simulink model "collectors"  (R2018a)
settings: Solver=VariableStepAuto  StartTime=0.0  StopTime=500  FixedStep=0.01  RelTol=1e-5
libraries: simulink x2
settings Model: Creator=daniel  LastModifiedBy=blond
settings SolverCC: ZeroCrossAlgorithm=Adaptive  AlgebraicLoopSolver=LineSearch
settings DebuggingCC: MaxConsecutiveZCsMsg=warning

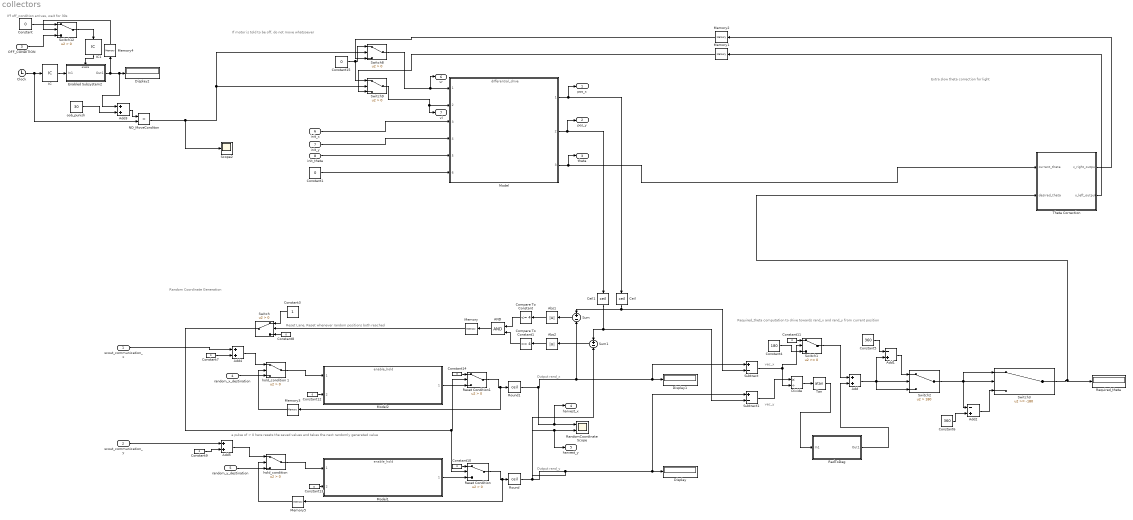
== system collectors ==
  note: If motor is told to be off, do not move whatsoever
  note: Extra slow theta correction for light
  note: Required_theta computation to drive towards rand_x and rand_y from current position
  note: vec_y
  note: Reset Lane, Reset whenever random positions both reached
  note: a pulse of > 0 here resets the saved values and takes the next randomly generated value
  note: Output rand_x
  note: Random Coordinate Generation
  note: Output rand_y
  note: vec_x
  note: Iff off_condition arrives, wait for 30s
  "scout_communication_x " : Inport
  scout_communication_y : Inport  Port=2
  "OFF_CONDITION " : Inport  Port=3  OutDataTypeStr=boolean
  random_x_destination : Inport  Port=4
  random_y_destination : Inport  Port=5
  "init_x " : Inport  Port=6
  init_y : Inport  Port=7
  "init_theta " : Inport  Port=8
  AND : Logic  IconShape=distinctive  AllPortsSameDT=off  OutDataTypeStr=boolean
  Abs1 : Abs
  Abs2 : Abs
  Add{,3..5} (4 alike) : Sum
  Add1 : Sum  Inputs=-+
  Add2 : Sum  Inputs=-+
  Ceil : Rounding  Operator=ceil
  Ceil1 : Rounding  Operator=ceil
  Clock : Clock
  Compare To Constant : simulink/Logic and Bit Operations/Compare To Constant  relop=<=  const=4  OutDataTypeStr=boolean
  Compare To Constant1 : simulink/Logic and Bit Operations/Compare To Constant  relop=<=  const=4  OutDataTypeStr=boolean
  Constant{,1,7..15} (11 alike) : Constant  Value=0
  Constant3 : Constant
  Constant4 : Constant  Value=180
  Constant5 : Constant  Value=360
  Constant6 : Constant  Value=360
  Display : Display
  Display1 : Display
  Display2 : Display
  Divide : Product  Inputs=*/
  Enabled Subsystem2 : Subsystem  TreatAsAtomicUnit=on
  IC : InitialCondition  Value=-30
  IC1 : InitialCondition
  Memory{,1..2,4} (4 alike) : Memory
  Memory3 : Memory  InheritSampleTime=on
  Memory5 : Memory  InheritSampleTime=on
  Model : ModelReference  ModelNameDialog=differential_drive.slx  SimulationMode=Normal  ModelReferenceVersion=1.313
  Model1 : ModelReference  ModelNameDialog=enable_hold.slx  SimulationMode=Normal  ModelReferenceVersion=1.286
  Model2 : ModelReference  ModelNameDialog=enable_hold.slx  SimulationMode=Normal  ModelReferenceVersion=1.286
  NO_MoveConditon : RelationalOperator  Operator=>  OutDataTypeStr=boolean  RndMeth=Simplest
  RadToDeg : Subsystem
  "RandomCoordinate Scope " : Scope  NumInputPorts=2
  Required_theta : Display
  Reset Condition : Switch  Criteria=u2 > Threshold
  Reset Condition1 : Switch  Criteria=u2 > Threshold
  Round : Rounding  Operator=ceil
  Round1 : Rounding  Operator=ceil
  Scope2 : Scope
  Subtract : Sum  Inputs=+-
  Subtract1 : Sum  Inputs=+-
  Sum : Sum  Inputs=+-
  Sum1 : Sum  Inputs=+-
  Switch{,8..9,12} (4 alike) : Switch  Criteria=u2 > Threshold
  Switch1 : Switch  ZeroCross=off
  Switch2 : Switch  Criteria=u2 > Threshold  Threshold=180  ZeroCross=off
  Switch3 : Switch  Threshold=-180  ZeroCross=off
  Tan : Trigonometry  Operator=atan  OutputSignalType=real
  "Theta Correction " : Subsystem
  "hold_condition " : Switch  Criteria=u2 > Threshold
  hold_condition 1 : Switch  Criteria=u2 > Threshold
  oob_punish : Constant  Value=30
  pos_x : Outport
  pos_y : Outport  Port=2
  theta : Outport  Port=3
  harvest_x : Outport  Port=4
  harvest_y : Outport  Port=5
  vr : Outport  Port=6
  vl : Outport  Port=7
  wires:
  "init_theta "/1 -> Model/5
  Model/1 -> pos_x/1, Ceil/1
  Model/2 -> pos_y/1, Ceil1/1
  Model/3 -> theta/1, "Theta Correction "/1(current_theta)
  Constant1/1 -> Model/6
  random_y_destination/1 -> "hold_condition "/3
  "hold_condition "/1 -> Model1/1
  Round/1 -> harvest_y/1, "RandomCoordinate Scope "/2, Sum1/2, Subtract1/1, Display/1
  Model1/1 -> Reset Condition/3
  Round1/1 -> harvest_x/1, "RandomCoordinate Scope "/1, Subtract/1, Display1/1, Sum/2
  Model2/1 -> Reset Condition1/3
  hold_condition 1/1 -> Model2/1
  random_x_destination/1 -> hold_condition 1/3
  Compare To Constant/1 -> AND/1
  Compare To Constant1/1 -> AND/2
  Ceil1/1 -> Sum1/1, Subtract1/2
  Ceil/1 -> Sum/1, Subtract/2
  AND/1 -> Memory/1
  Constant3/1 -> Switch/1
  Memory/1 -> Switch/2
  Switch/1 -> Reset Condition/2, Reset Condition1/2
  Subtract1/1 -> Divide/1
  Subtract/1 -> Switch1/2, Divide/2
  Divide/1 -> Tan/1
  Tan/1 -> RadToDeg/1(In1)
  Switch1/1 -> Add/1
  Constant4/1 -> Switch1/3
  Add/1 -> Switch2/3, Switch2/2, Add1/2
  Constant5/1 -> Add1/1
  Add1/1 -> Switch2/1
  Switch2/1 -> Switch3/1, Switch3/2, Add2/1
  Constant6/1 -> Add2/2
  Add2/1 -> Switch3/3
  Switch3/1 -> "Theta Correction "/2(desired_theta), Required_theta/1
  RadToDeg/1(Out1) -> Add/2
  Constant7/1 -> Add4/2
  Constant8/1 -> Switch/3
  Constant10/1 -> Reset Condition/1
  Constant11/1 -> Switch1/1
  Constant12/1 -> Model2/2
  Constant13/1 -> Model1/2
  Constant14/1 -> Reset Condition1/1
  Reset Condition1/1 -> Memory3/1, Round1/1
  Reset Condition/1 -> Memory5/1, Round/1
  Sum/1 -> Abs1/1
  Abs1/1 -> Compare To Constant/1
  Abs2/1 -> Compare To Constant1/1
  Sum1/1 -> Abs2/1
  Memory5/1 -> "hold_condition "/2
  Memory3/1 -> hold_condition 1/2
  Add4/1 -> hold_condition 1/1
  Constant9/1 -> Add5/2
  Add5/1 -> "hold_condition "/1
  "scout_communication_x "/1 -> Add4/1
  scout_communication_y/1 -> Add5/1
  Constant15/1 -> Switch9/1, Switch8/1
  Switch8/1 -> vr/1, Model/1
  Switch9/1 -> vl/1, Model/2
  "init_x "/1 -> Model/3
  init_y/1 -> Model/4
  Memory1/1 -> Switch9/3
  Memory2/1 -> Switch8/3
  "Theta Correction "/2(v_left_output) -> Memory1/1
  "Theta Correction "/1(v_right_output) -> Memory2/1
  "OFF_CONDITION "/1 -> Switch12/3
  NO_MoveConditon/1 -> Scope2/1, Switch9/2, Switch8/2
  oob_punish/1 -> Add3/2
  Add3/1 -> NO_MoveConditon/1
  Enabled Subsystem2/1(Out1) -> Memory4/1, Add3/1, Display2/1
  Clock/1 -> NO_MoveConditon/2, IC/1
  Switch12/1 -> IC1/1
  Memory4/1 -> Switch12/2
  IC1/1 -> Enabled Subsystem2/Enable
  IC/1 -> Enabled Subsystem2/1(In1)
  Constant/1 -> Switch12/1

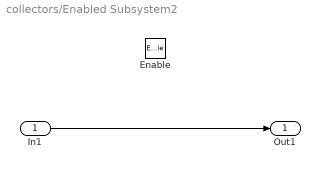
== system collectors/Enabled Subsystem2 ==
  In1 : Inport
  Enable : EnablePort
  Out1 : Outport
  wires:
  In1/1 -> Out1/1

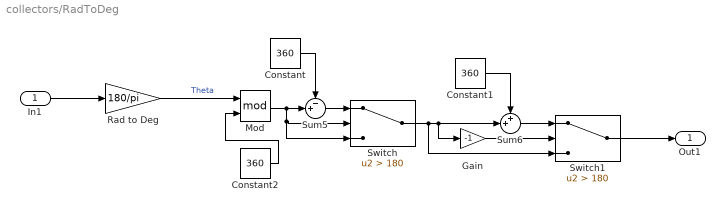
== system collectors/RadToDeg ==
  In1 : Inport
  Constant : Constant  Value=360
  Constant1 : Constant  Value=360
  Constant2 : Constant  Value=360
  Gain : Gain  Gain=-1
  Mod : Math  Operator=mod  SaturateOnIntegerOverflow=on
  Rad to Deg : Gain  Gain=180/pi
  Sum5 : Sum  Inputs=-+|
  Sum6 : Sum  Inputs=++|
  Switch : Switch  Criteria=u2 > Threshold  Threshold=180
  Switch1 : Switch  Criteria=u2 > Threshold  Threshold=180
  Out1 : Outport
  wires:
  Constant/1 -> Sum5/1
  Constant1/1 -> Sum6/1
  Rad to Deg/1 -> Mod/1  "Theta"
  Gain/1 -> Switch1/2
  Switch/1 -> Sum6/2, Gain/1, Switch1/3
  Sum5/1 -> Switch/1
  Mod/1 -> Sum5/2, Switch/2, Switch/3
  Sum6/1 -> Switch1/1
  Constant2/1 -> Mod/2
  In1/1 -> Rad to Deg/1
  Switch1/1 -> Out1/1

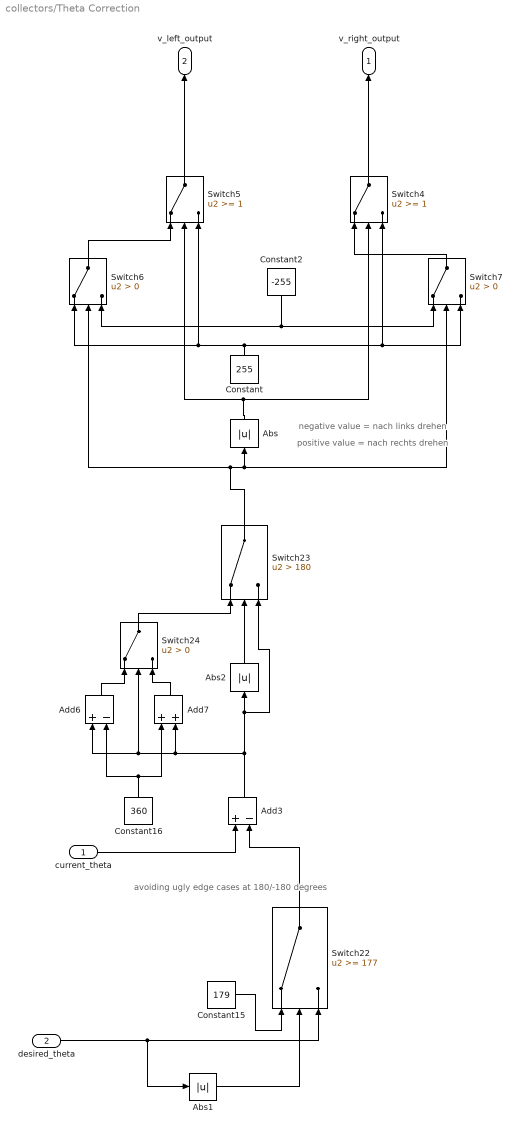
== system collectors/Theta Correction  ==
  note: avoiding ugly edge cases at
      | 180/-180 degrees
  note: positive value = nach rechts drehen
  note: negative value = nach links drehen
  current_theta : Inport
  desired_theta : Inport  Port=2
  Abs : Abs  ZeroCross=off
  Abs1 : Abs  ZeroCross=off
  Abs2 : Abs  ZeroCross=off
  Add3 : Sum  Inputs=+-
  Add6 : Sum  Inputs=+-
  Add7 : Sum
  Constant : Constant  Value=255
  Constant15 : Constant  Value=179
  Constant16 : Constant  Value=360
  Constant2 : Constant  Value=-255
  Switch22 : Switch  Threshold=177  ZeroCross=off
  Switch23 : Switch  Criteria=u2 > Threshold  Threshold=180  ZeroCross=off
  Switch24 : Switch  Criteria=u2 > Threshold  ZeroCross=off
  Switch4 : Switch  Threshold=1  ZeroCross=off
  Switch5 : Switch  Threshold=1  ZeroCross=off
  Switch6 : Switch  Criteria=u2 > Threshold  ZeroCross=off
  Switch7 : Switch  Criteria=u2 > Threshold  ZeroCross=off
  v_right_output : Outport
  v_left_output : Outport  Port=2
  wires:
  desired_theta/1 -> Switch22/3, Abs1/1
  current_theta/1 -> Add3/1
  Switch5/1 -> v_left_output/1
  Switch6/1 -> Switch5/1
  Switch7/1 -> Switch4/1
  Abs/1 -> Switch4/2, Switch5/2
  Constant2/1 -> Switch7/1, Switch6/3
  Switch23/1 -> Abs/1, Switch7/2, Switch6/2
  Constant/1 -> Switch7/3, Switch4/3, Switch6/1, Switch5/3
  Switch4/1 -> v_right_output/1
  Abs1/1 -> Switch22/2
  Switch22/1 -> Add3/2
  Constant15/1 -> Switch22/1
  Add3/1 -> Add7/2, Add6/1, Switch24/2, Switch23/3, Abs2/1
  Abs2/1 -> Switch23/2
  Add6/1 -> Switch24/1
  Constant16/1 -> Add6/2, Add7/1
  Add7/1 -> Switch24/3
  Switch24/1 -> Switch23/1
